simulink model "systolic_hwcosim"  (R2021a)
settings: Solver=VariableStepAuto  StartTime=0.0  StopTime=100  RelTol=1e-3
undefined symbols (not defined in the file or in its folder): A, N
libraries: hdlBasic x30, pelib x16, xbsIndex_r4 x1, JTAGRuntimeCosim_r4 x1
settings Model: Creator=asc8  LastModifiedBy=asc8

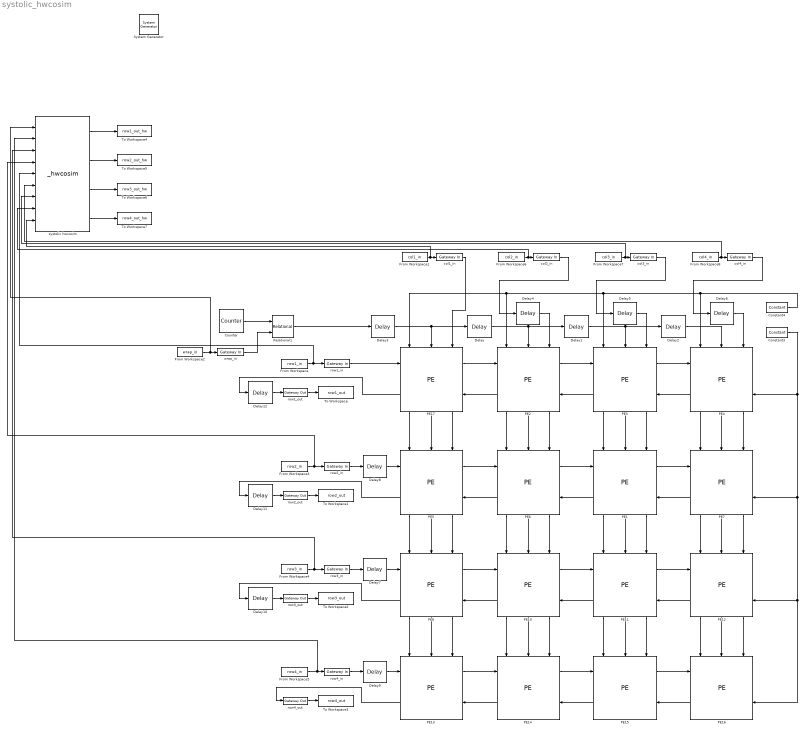
== system systolic_hwcosim ==
  " System Generator" : xbsIndex_r4/ System Generator  Tag=genX  xilinxfamily=zynq  part=xc7z020  speed=-1  package=clg484  synthesis_tool=Vivado  clock_wrapper=Clock Enables  directory=./netlist  proj_type=Vivado  Synth_file=Vivado Synthesis Defaults  Impl_file=Vivado Implementation Defaults  testbench=off  simulink_period=1  sysclk_period=2.75  dcm_input_clock_period=10  incr_netlist=off  trim_vbits=Everywhere in SubSystem  dbl_ovrd=According to Block Masks  core_generation=According to Block Masks  run_coregen=off  deprecated_control=off  eval_field=0  block_type=sysgen
  Constant3 : hdlBasic/Constant  const=0  gui_display_data_type=Fixed-point  arith_type=Signed (2's comp)  n_bits=16  bin_pt=0  preci_type=Single  exp_width=8  frac_width=24  explicit_period=on  period=1  XmcBlockStatus=1  maskContainerNames=tabcontainer1  block_type=constant  block_config=sysgen:Constant_config
  Constant4 : hdlBasic/Constant  const=1  gui_display_data_type=Boolean  arith_type=Boolean  n_bits=16  bin_pt=0  preci_type=Single  exp_width=8  frac_width=24  explicit_period=on  period=1  XmcBlockStatus=1  maskContainerNames=tabcontainer1  block_type=constant  block_config=sysgen:Constant_config
  Counter : hdlBasic/Counter  cnt_type=Count limited  cnt_to=3  operation=Up  start_count=0  cnt_by_val=1  arith_type=Unsigned  n_bits=2  bin_pt=0  load_pin=off  rst=off  en=off  explicit_period=Explicit  period=1  use_behavioral_HDL=off  implementation=Fabric  XmcBlockStatus=1  maskContainerNames=group1  block_type=counter  block_config=sysgen:Counter_config
  Delay{,1..2,4,8,10} (6 alike) : hdlBasic/Delay  rst=off  en=off  latency=1  reg_retiming=off  XmcBlockStatus=1  maskContainerNames=group1  block_type=delay  block_config=sysgen:Delay_config
  Delay{3,5,7,11} (4 alike) : hdlBasic/Delay  rst=off  en=off  latency=2  reg_retiming=off  XmcBlockStatus=1  maskContainerNames=group1  block_type=delay  block_config=sysgen:Delay_config
  Delay12 : hdlBasic/Delay  rst=off  en=off  latency=3  reg_retiming=off  XmcBlockStatus=1  maskContainerNames=group1  block_type=delay  block_config=sysgen:Delay_config
  Delay6 : hdlBasic/Delay  rst=off  en=off  latency=3  reg_retiming=off  XmcBlockStatus=1  maskContainerNames=group1  block_type=delay  block_config=sysgen:Delay_config
  Delay9 : hdlBasic/Delay  rst=off  en=off  latency=3  reg_retiming=off  XmcBlockStatus=1  maskContainerNames=group1  block_type=delay  block_config=sysgen:Delay_config
  From Workspace : FromWorkspace  VariableName=row1_in
  From Workspace1 : FromWorkspace  VariableName=col1_in
  From Workspace2 : FromWorkspace  VariableName=wrap_in
  From Workspace3 : FromWorkspace  VariableName=row2_in
  From Workspace4 : FromWorkspace  VariableName=row3_in
  From Workspace5 : FromWorkspace  VariableName=row4_in
  From Workspace6 : FromWorkspace  VariableName=col2_in
  From Workspace7 : FromWorkspace  VariableName=col3_in
  From Workspace8 : FromWorkspace  VariableName=col4_in
  PE{1..8,10..17} (16 alike) : pelib/PE  SystemSampleTime=-1  VariantActivationTime=update diagram  Latency=0  AutoFrameSizeCalculation=off
      settings: SourceProductName=Aedan's PE Library  PortSchema="{\"entries\":[{\"content\":{\"sides\":[{\"content\":{\"connectorIds\":[\"In1\",\"Out5\"]},\"type\":\"ConnectorPlacement.EquallySpacedRectSide\",\"uuid\":\"f7e55443-70fb-4ed5-ab4f-147f7311106a\"},{\"content\":{\"connectorIds\":[\"Out1\",\"In5\"],\"side\":\"RIGHT\"},\"type\":\"ConnectorPlacement.EquallySpacedRectSide\",\"uuid\":\"6de0769a-4a22-4abb-b630-26d0c175204f\"},{\"content\":{\"connectorIds\":[\"In2\",\"In3\",\"In4\"],\"side\":\"TOP\"},\"type\":\"ConnectorPlacement.EquallySpacedRectSide\",\"uuid\":\"a041cc58-78e8-4444-b053-dd6f2c27badd\"},{\"content\":{\"connectorIds\":[\"Out2\",\"Out3\",\"Out4\"],\"side\":\"BOTTOM\"},\"type\":\"ConnectorPlacement.EquallySpacedRectSide\",\"uuid\":\"085ff6f5-8624-4aab-b622-9beedcd77ebd\"}]},\"type\":\"ConnectorPlacement.EquallySpacedConnector\",\"uuid\":\"928950cd-8b9e-4ebf-b8fd-b98c3e494fdc\"}],\"packageUris\":[\"http://schema.mathworks.com/mf0/Connector/R2020b\"],\"version\":\"1.0\"}"
  Relational1 : hdlBasic/Relational  mode=a=b  op_type=Bool  en=off  latency=0  XmcBlockStatus=1  maskContainerNames=tabcontainer1  block_type=relational  block_config=sysgen:Relational_config
  To Workspace : ToWorkspace  VariableName=row1_out  SaveFormat=Timeseries  SampleTime=-1
  To Workspace1 : ToWorkspace  VariableName=row2_out  SaveFormat=Timeseries  SampleTime=-1
  To Workspace2 : ToWorkspace  VariableName=row3_out  SaveFormat=Timeseries  SampleTime=-1
  To Workspace3 : ToWorkspace  VariableName=row4_out  SaveFormat=Timeseries  SampleTime=-1
  To Workspace4 : ToWorkspace  VariableName=row1_out_hw  SaveFormat=Timeseries  SampleTime=-1
  To Workspace5 : ToWorkspace  VariableName=row2_out_hw  SaveFormat=Timeseries  SampleTime=-1
  To Workspace6 : ToWorkspace  VariableName=row3_out_hw  SaveFormat=Timeseries  SampleTime=-1
  To Workspace7 : ToWorkspace  VariableName=row4_out_hw  SaveFormat=Timeseries  SampleTime=-1
  col1_in : hdlBasic/Gateway In  gui_display_data_type=Fixed-point  arith_type=Signed (2's comp)  n_bits=16  bin_pt=0  preci_type=Single  exp_width=8  frac_width=24  rows=1  columns=1  quantization="Round  (unbiased: +/- Inf)"  overflow=Saturate  period=1  UseAsADC=off  ADCChannel='1'  interface=None  automatic_assignment=on  address_offset=hex2dec('00')  intf_name=''  intf_description=''  default_value=0  timing_constraint=None  locs_specified=off  LOCs={}  io_standard={}  inherit_from_input=off  hdl_port=on  XmcBlockStatus=1  maskContainerNames=group4  block_type=gatewayin  block_config=sysgen:gateway_in_config  block_width_w=590  block_height_w=620  block_width=640  block_height=850
  col2_in : hdlBasic/Gateway In  gui_display_data_type=Fixed-point  arith_type=Signed (2's comp)  n_bits=16  bin_pt=0  preci_type=Single  exp_width=8  frac_width=24  rows=1  columns=1  quantization="Round  (unbiased: +/- Inf)"  overflow=Saturate  period=1  UseAsADC=off  ADCChannel='1'  interface=None  automatic_assignment=on  address_offset=hex2dec('00')  intf_name=''  intf_description=''  default_value=0  timing_constraint=None  locs_specified=off  LOCs={}  io_standard={}  inherit_from_input=off  hdl_port=on  XmcBlockStatus=1  maskContainerNames=group4  block_type=gatewayin  block_config=sysgen:gateway_in_config  block_width_w=590  block_height_w=620  block_width=640  block_height=850
  col3_in : hdlBasic/Gateway In  gui_display_data_type=Fixed-point  arith_type=Signed (2's comp)  n_bits=16  bin_pt=0  preci_type=Single  exp_width=8  frac_width=24  rows=1  columns=1  quantization="Round  (unbiased: +/- Inf)"  overflow=Saturate  period=1  UseAsADC=off  ADCChannel='1'  interface=None  automatic_assignment=on  address_offset=hex2dec('00')  intf_name=''  intf_description=''  default_value=0  timing_constraint=None  locs_specified=off  LOCs={}  io_standard={}  inherit_from_input=off  hdl_port=on  XmcBlockStatus=1  maskContainerNames=group4  block_type=gatewayin  block_config=sysgen:gateway_in_config  block_width_w=590  block_height_w=620  block_width=640  block_height=850
  col4_in : hdlBasic/Gateway In  gui_display_data_type=Fixed-point  arith_type=Signed (2's comp)  n_bits=16  bin_pt=0  preci_type=Single  exp_width=8  frac_width=24  rows=1  columns=1  quantization="Round  (unbiased: +/- Inf)"  overflow=Saturate  period=1  UseAsADC=off  ADCChannel='1'  interface=None  automatic_assignment=on  address_offset=hex2dec('00')  intf_name=''  intf_description=''  default_value=0  timing_constraint=None  locs_specified=off  LOCs={}  io_standard={}  inherit_from_input=off  hdl_port=on  XmcBlockStatus=1  maskContainerNames=group4  block_type=gatewayin  block_config=sysgen:gateway_in_config  block_width_w=590  block_height_w=620  block_width=640  block_height=850
  row1_in : hdlBasic/Gateway In  gui_display_data_type=Fixed-point  arith_type=Signed (2's comp)  n_bits=16  bin_pt=0  preci_type=Single  exp_width=8  frac_width=24  rows=1  columns=1  quantization="Round  (unbiased: +/- Inf)"  overflow=Saturate  period=1  UseAsADC=off  ADCChannel='1'  interface=None  automatic_assignment=on  address_offset=hex2dec('00')  intf_name=''  intf_description=''  default_value=0  timing_constraint=None  locs_specified=off  LOCs={}  io_standard={}  inherit_from_input=off  hdl_port=on  XmcBlockStatus=1  maskContainerNames=group4  block_type=gatewayin  block_config=sysgen:gateway_in_config  block_width_w=590  block_height_w=620  block_width=640  block_height=850
  row1_out : hdlBasic/Gateway Out  inherit_from_input=off  hdl_port=on  rows=1  columns=1  UseAsDAC=off  DACChannel='1'  interface=None  automatic_assignment=on  address_offset=hex2dec('00')  intf_name=''  intf_description=''  timing_constraint=None  locs_specified=off  LOCs={}  io_standard={}  XmcBlockStatus=1  maskContainerNames=group4  block_type=gatewayout  block_config=sysgen:gateway_out_config  block_width_w=590  block_height_w=620  block_width=620  block_height=750
  row2_in : hdlBasic/Gateway In  gui_display_data_type=Fixed-point  arith_type=Signed (2's comp)  n_bits=16  bin_pt=0  preci_type=Single  exp_width=8  frac_width=24  rows=1  columns=1  quantization="Round  (unbiased: +/- Inf)"  overflow=Saturate  period=1  UseAsADC=off  ADCChannel='1'  interface=None  automatic_assignment=on  address_offset=hex2dec('00')  intf_name=''  intf_description=''  default_value=0  timing_constraint=None  locs_specified=off  LOCs={}  io_standard={}  inherit_from_input=off  hdl_port=on  XmcBlockStatus=1  maskContainerNames=group4  block_type=gatewayin  block_config=sysgen:gateway_in_config  block_width_w=590  block_height_w=620  block_width=640  block_height=850
  row2_out : hdlBasic/Gateway Out  inherit_from_input=off  hdl_port=on  rows=1  columns=1  UseAsDAC=off  DACChannel='1'  interface=None  automatic_assignment=on  address_offset=hex2dec('00')  intf_name=''  intf_description=''  timing_constraint=None  locs_specified=off  LOCs={}  io_standard={}  XmcBlockStatus=1  maskContainerNames=group4  block_type=gatewayout  block_config=sysgen:gateway_out_config  block_width_w=590  block_height_w=620  block_width=620  block_height=750
  row3_in : hdlBasic/Gateway In  gui_display_data_type=Fixed-point  arith_type=Signed (2's comp)  n_bits=16  bin_pt=0  preci_type=Single  exp_width=8  frac_width=24  rows=1  columns=1  quantization="Round  (unbiased: +/- Inf)"  overflow=Saturate  period=1  UseAsADC=off  ADCChannel='1'  interface=None  automatic_assignment=on  address_offset=hex2dec('00')  intf_name=''  intf_description=''  default_value=0  timing_constraint=None  locs_specified=off  LOCs={}  io_standard={}  inherit_from_input=off  hdl_port=on  XmcBlockStatus=1  maskContainerNames=group4  block_type=gatewayin  block_config=sysgen:gateway_in_config  block_width_w=590  block_height_w=620  block_width=640  block_height=850
  row3_out : hdlBasic/Gateway Out  inherit_from_input=off  hdl_port=on  rows=1  columns=1  UseAsDAC=off  DACChannel='1'  interface=None  automatic_assignment=on  address_offset=hex2dec('00')  intf_name=''  intf_description=''  timing_constraint=None  locs_specified=off  LOCs={}  io_standard={}  XmcBlockStatus=1  maskContainerNames=group4  block_type=gatewayout  block_config=sysgen:gateway_out_config  block_width_w=590  block_height_w=620  block_width=620  block_height=750
  row4_in : hdlBasic/Gateway In  gui_display_data_type=Fixed-point  arith_type=Signed (2's comp)  n_bits=16  bin_pt=0  preci_type=Single  exp_width=8  frac_width=24  rows=1  columns=1  quantization="Round  (unbiased: +/- Inf)"  overflow=Saturate  period=1  UseAsADC=off  ADCChannel='1'  interface=None  automatic_assignment=on  address_offset=hex2dec('00')  intf_name=''  intf_description=''  default_value=0  timing_constraint=None  locs_specified=off  LOCs={}  io_standard={}  inherit_from_input=off  hdl_port=on  XmcBlockStatus=1  maskContainerNames=group4  block_type=gatewayin  block_config=sysgen:gateway_in_config  block_width_w=590  block_height_w=620  block_width=640  block_height=850
  row4_out : hdlBasic/Gateway Out  inherit_from_input=off  hdl_port=on  rows=1  columns=1  UseAsDAC=off  DACChannel='1'  interface=None  automatic_assignment=on  address_offset=hex2dec('00')  intf_name=''  intf_description=''  timing_constraint=None  locs_specified=off  LOCs={}  io_standard={}  XmcBlockStatus=1  maskContainerNames=group4  block_type=gatewayout  block_config=sysgen:gateway_out_config  block_width_w=590  block_height_w=620  block_width=620  block_height=750
  systolic hwcosim : JTAGRuntimeCosim_r4/_hwcosim  clkSrc=Single Stepped  hasCombinationalPath=on  bitfileName=C:\ELEC522\asc8\prj2\netlist\systolic.bit  skipConfig=off  dispPartInfo=off  useZynqReconfigScript=on  cable=Auto Detect  speed=N/A  cablePort=N/A  cableLocation=Local  shareCable=off  xmp=[]  software_settings=[]  design_xtable=|  binDir=[]  engineDll=JTAGCosimEngine.dll  cableWaitTime=10  bscanPos=-1  IRLengths=[]  useWaitBox=1  hasBufgmux=on  Scheme=Cosim  useCmdProc=1  hasProc=0  useImpact=0  printLogFile=0  userChain=2  XmcBlockStatus=0  maskContainerNames=tabcontainer1  block_type=jtagcosim  block_config=Sysgen:hwcosim_block_config
      | {
      |     'clkWrapper' => 'systolic',
      |     'burstMode' => false,
      |     'burstFifoDepth' => '1024',
      |     'shared_memories' => {},
      |     'clocksGcd' => 1,
      |     'device' => {
      |       'family' => 'zynq',
      |       'part' => 'xc7z020',
      |       'package' => 'clg484',
      |       'speed' => '-1',
      |     },
      |     'ports' => {
      |       'wrap_in' => {
      |         'direction' => 'in',
      |         'width' => 2,
      |         'name' => 'wrap_in',
      |         'period' => 1,
      |         'icon_text' => 'wrap_in',
      |         'type' => 'UFix_2_0',
      |         'arithmetic_type' => 'xlUnsigned',
      |         'dat_file' => 'systolic_wrap_in.dat',
      |         'bin_pt' => 0,
      |         'addr_offset' => 0,
      |         'bd_port_index' => 0,
      |       },
      |       'row4_in' => {
      |         'direction' => 'in',
      |         'width' => 16,
      |         'name' => 'row4_in',
      |         'period' => 1,
      |         'icon_text' => 'row4_in',
      |         'type' => 'Fix_16_0',
      |         'arithmetic_type' => 'xlSigned',
      |         'dat_file' => 'systolic_row4_in.dat',
      |         'bin_pt' => 0,
      |         'addr_offset' => 4,
      |         'bd_port_index' => 1,
      |       },
      |       'row3_in' => {
      |         'direction' => 'in',
      |         'width' => 16,
      |         'name' => 'row3_in',
      |         'period' => 1,
      |         'icon_text' => 'row3_in',
      |         'type' => 'Fix_16_0',
      |         'arithmetic_type' => 'xlSigned',
      |         'dat_file' => 'systolic_row3_in.dat',
      |         'bin_pt' => 0,
      |         'addr_offset' => 8,
      |         'bd_port_index' => 2,
      |       },
      |       'row2_in' => {
      |         'direction' => 'in',
      |         'width' => 16,
      |         'name' => 'row2_in',
      |         'period' => 1,
      |         'icon_text' => 'row2_in',
      |         'type' => 'Fix_16_0',
      |         'arithmetic_type' => 'xlSigned',
      |         'dat_file' => 'systolic_row2_in.dat',
      |         'bin_pt' => 0,
      |         'addr_offset' => 12,
      |         'bd_port_index' => 3,
      |       },
      |       'row1_in' => {
      |         'direction' => 'in',
      |         'width' => 16,
      |         'name' => 'row1_in',
      |         'period' => 1,
      |         'icon_text' => 'row1_in',
      |         'type' => 'Fix_16_0',
      |         'arithmetic_type' => 'xlSigned',
      |         'dat_file' => 'systolic_row1_in.dat',
      |         'bin_pt' => 0,
      |         'addr_offset' => 16,
      |         'bd_port_index' => 4,
      |       },
      |       'col4_in' => {
      |         'direction' => 'in',
      |         'width' => 16,
      |         'name' => 'col4_in',
      |         'period' => 1,
      |         'icon_text' => 'col4_in',
      |         'type' => 'Fix_16_0',
      |         'arithmetic_type' => 'xlSigned',
      |         'dat_file' => 'systolic_col4_in.dat',
      |         'bin_pt' => 0,
      |         'addr_offset' => 20,
      |         'bd_port_index' => 5,
      |       },
      |       'col3_in' => {
      |         'direction' => 'in',
      |         'width' => 16,
      |         'name' => 'col3_in',
      |         'period' => 1,
      |         'icon_text' => 'col3_in',
      |         'type' => 'Fix_16_0',
      |         'arithmetic_type' => 'xlSigned',
      |         'dat_file' => 'systolic_col3_in.dat',
      |         'bin_pt' => 0,
      |         'addr_offset' => 24,
      |         'bd_port_index' => 6,
      |       },
      |       'col2_in' => {
      |         'direction' => 'in',
      |         'width' => 16,
      |         'name' => 'col2_in',
      |         'period' => 1,
      |         'icon_text' => 'col2_in',
      |         'type' => 'Fix_16_0',
      |         'arithmetic_type' => 'xlSigned',
      |         'dat_file' => 'systolic_col2_in.dat',
      |         'bin_pt' => 0,
      |         'addr_offset' => 28,
      |         'bd_port_index' => 7,
      |       },
      |       'col1_in' => {
      |         'direction' => 'in',
      |         'width' => 16,
      |         'name' => 'col1_in',
      |         'period' => 1,
      |         'icon_text' => 'col1_in',
      |         'type' => 'Fix_16_0',
      |         'arithmetic_type' => 'xlSigned',
      |         'dat_file' => 'systolic_col1_in.dat',
      |         'bin_pt' => 0,
      |         'addr_offset' => 32,
      |         'bd_port_index' => 8,
      |       },
      |       'row1_out' => {
      |         'direction' => 'out',
      |         'width' => 16,
      |         'name' => 'row1_out',
      |         'period' => 1,
      |         'icon_text' => 'row1_out',
      |         'type' => 'Fix_16_0',
      |         'arithmetic_type' => 'xlSigned',
      |         'dat_file' => 'systolic_row1_out.dat',
      |         'bin_pt' => 0,
      |         'addr_offset' => 36,
      |         'bd_port_index' => 0,
      |       },
      |       'row2_out' => {
      |         'direction' => 'out',
      |         'width' => 16,
      |         'name' => 'row2_out',
      |         'period' => 1,
      |         'icon_text' => 'row2_out',
      |         'type' => 'Fix_16_0',
      |         'arithmetic_type' => 'xlSigned',
      |         'dat_file' => 'systolic_row2_out.dat',
      |         'bin_pt' => 0,
      |         'addr_offset' => 40,
      |         'bd_port_index' => 1,
      |       },
      |       'row3_out' => {
      |         'direction' => 'out',
      |         'width' => 16,
      |         'name' => 'row3_out',
      |         'period' => 1,
      |         'icon_text' => 'row3_out',
      |         'type' => 'Fix_16_0',
      |         'arithmetic_type' => 'xlSigned',
      |         'dat_file' => 'systolic_row3_out.dat',
      |         'bin_pt' => 0,
      |         'addr_offset' => 44,
      |         'bd_port_index' => 2,
      |       },
      |       'row4_out' => {
      |         'direction' => 'out',
      |         'width' => 16,
      |         'name' => 'row4_out',
      |         'period' => 1,
      |         'icon_text' => 'row4_out',
      |         'type' => 'Fix_16_0',
      |         'arithmetic_type' => 'xlSigned',
      |         'dat_file' => 'systolic_row4_out.dat',
      |         'bin_pt' => 0,
      |         'addr_offset' => 48,
      |         'bd_port_index' => 3,
      |       },
      |     },
      |   }
  wrap_in : hdlBasic/Gateway In  gui_display_data_type=Fixed-point  arith_type=Unsigned  n_bits=2  bin_pt=0  preci_type=Single  exp_width=8  frac_width=24  rows=1  columns=1  quantization="Round  (unbiased: +/- Inf)"  overflow=Saturate  period=1  UseAsADC=off  ADCChannel='1'  interface=None  automatic_assignment=on  address_offset=hex2dec('00')  intf_name=''  intf_description=''  default_value=0  timing_constraint=None  locs_specified=off  LOCs={}  io_standard={}  inherit_from_input=off  hdl_port=on  XmcBlockStatus=1  maskContainerNames=group4  block_type=gatewayin  block_config=sysgen:gateway_in_config  block_width_w=590  block_height_w=620  block_width=640  block_height=850
  wires:
  PE11/2 -> PE15/2
  PE4/2 -> PE7/2
  PE3/1 -> PE4/1
  Delay1/1 -> Delay2/1, PE3/3
  PE3/2 -> PE1/2
  PE7/2 -> PE12/2
  PE4/4 -> PE7/4
  PE1/1 -> PE7/1
  PE2/2 -> PE6/2
  PE15/5 -> PE14/5
  PE1/2 -> PE11/2
  PE2/5 -> PE17/5
  PE1/3 -> PE11/3
  PE3/4 -> PE1/4
  PE8/3 -> PE13/3
  PE15/1 -> PE16/1
  PE14/1 -> PE15/1
  PE10/1 -> PE11/1
  PE6/2 -> PE10/2
  Constant3/1 -> PE4/5, PE7/5, PE12/5, PE16/5
  PE6/3 -> PE10/3
  PE11/5 -> PE10/5
  PE3/5 -> PE2/5
  PE4/3 -> PE7/3
  PE5/3 -> PE8/3
  PE17/4 -> PE5/4
  PE5/1 -> PE6/1
  PE11/3 -> PE15/3
  PE13/1 -> PE14/1
  PE6/4 -> PE10/4
  PE8/4 -> PE13/4
  PE11/1 -> PE12/1
  PE10/5 -> PE8/5
  PE10/4 -> PE14/4
  PE11/4 -> PE15/4
  PE12/2 -> PE16/2
  PE10/2 -> PE14/2
  PE12/4 -> PE16/4
  PE10/3 -> PE14/3
  PE12/3 -> PE16/3
  PE17/2 -> PE5/2
  PE5/2 -> PE8/2
  PE16/5 -> PE15/5
  PE4/5 -> PE3/5
  PE2/3 -> PE6/3
  PE1/4 -> PE11/4
  PE12/5 -> PE11/5
  PE7/4 -> PE12/4
  PE5/4 -> PE8/4
  PE2/1 -> PE3/1
  PE17/3 -> PE5/3
  Delay/1 -> Delay1/1, PE2/3
  PE14/5 -> PE13/5
  PE1/5 -> PE6/5
  PE17/1 -> PE2/1
  PE8/1 -> PE10/1
  PE2/4 -> PE6/4
  PE7/3 -> PE12/3
  PE7/5 -> PE1/5
  PE6/1 -> PE1/1
  PE8/2 -> PE13/2
  PE3/3 -> PE1/3
  PE6/5 -> PE5/5
  Delay2/1 -> PE4/3
  Counter/1 -> Relational1/1
  From Workspace/1 -> systolic hwcosim/5, row1_in/1
  row1_out/1 -> To Workspace/1
  From Workspace1/1 -> systolic hwcosim/9, col1_in/1
  col1_in/1 -> PE17/4
  From Workspace3/1 -> systolic hwcosim/4, row2_in/1
  row2_out/1 -> To Workspace1/1
  From Workspace4/1 -> systolic hwcosim/3, row3_in/1
  row3_out/1 -> To Workspace2/1
  From Workspace5/1 -> systolic hwcosim/2, row4_in/1
  PE13/5 -> row4_out/1
  row4_out/1 -> To Workspace3/1
  From Workspace6/1 -> systolic hwcosim/8, col2_in/1
  From Workspace7/1 -> systolic hwcosim/7, col3_in/1
  From Workspace8/1 -> systolic hwcosim/6, col4_in/1
  Delay3/1 -> PE17/3, Delay/1
  Relational1/1 -> Delay3/1
  Delay4/1 -> PE2/4
  col2_in/1 -> Delay4/1
  Delay5/1 -> PE3/4
  col3_in/1 -> Delay5/1
  Delay6/1 -> PE4/4
  col4_in/1 -> Delay6/1
  row1_in/1 -> PE17/1
  Delay8/1 -> PE5/1
  row2_in/1 -> Delay8/1
  Delay7/1 -> PE8/1
  row3_in/1 -> Delay7/1
  row4_in/1 -> Delay9/1
  Delay9/1 -> PE13/1
  PE8/5 -> Delay10/1
  Delay10/1 -> row3_out/1
  Delay11/1 -> row2_out/1
  PE5/5 -> Delay11/1
  Delay12/1 -> row1_out/1
  PE17/5 -> Delay12/1
  wrap_in/1 -> Relational1/2
  Constant4/1 -> PE17/2, PE2/2, PE3/2, PE4/2
  systolic hwcosim/1 -> To Workspace4/1
  systolic hwcosim/2 -> To Workspace5/1
  systolic hwcosim/3 -> To Workspace6/1
  systolic hwcosim/4 -> To Workspace7/1
  From Workspace2/1 -> systolic hwcosim/1, wrap_in/1
